simulink model "OPCModel"  (R2021a)
settings: Solver=VariableStepAuto  StartTime=0.0  StopTime=10.0  RelTol=1e-3
values from neighbouring files (symbols this model uses):
  ih = 22    [Data.m]
  it = 30    [Data.m]
  rhd = 0.75    [Data.m]
  rtd = 0.5    [Data.m]
undefined symbols (not defined in the file or in its folder): Ts
settings Model: Creator=jpss8  LastModifiedBy=jpss8

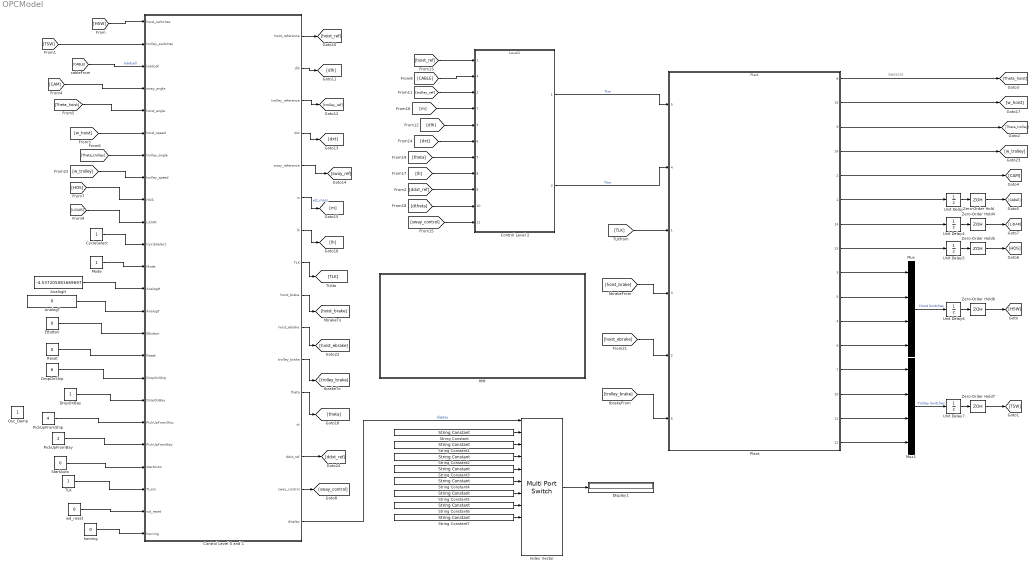
== system OPCModel ==
  note: Sensors
  AnalogH : Constant  Value=-4.537205081669697
  AnalogT : Constant  Value=0
  Control Level 0 and 1 : Subsystem
  Control Level 2 : ModelReference  ModelNameDialog=Level2.slx  SimulationMode=Normal  ModelReferenceVersion=1.293
      settings: PortSchema="{\"entries\":[{\"content\":{\"sides\":[{\"content\":{\"connectorIds\":[\"In1\",\"In4\",\"In2\",\"In7\",\"In3\",\"In6\",\"In5\",\"In8\",\"In9\",\"In10\",\"In11\"]},\"type\":\"ConnectorPlacement.EquallySpacedRectSide\",\"uuid\":\"5b552c0d-337f-40a2-963f-8f26f74218b0\"},{\"content\":{\"connectorIds\":[\"Out1\",\"Out2\"],\"side\":\"RIGHT\"},\"type\":\"ConnectorPlacement.EquallySpacedRectSide\",\"uuid\":\"4a33d29a-936e-4be9-945f-1937d64852b3\"},{\"content\":{\"connectorIds\":[],\"side\":\"TOP\"},\"type\":\"ConnectorPlacement.EquallySpacedRectSide\",\"uuid\":\"a706c8bd-7eef-4f34-a788-a1dec70d0973\"}]},\"type\":\"ConnectorPlacement.EquallySpacedConnector\",\"uuid\":\"61d5689b-6159-4c49-bed6-a66cde254875\"}],\"packageUris\":[\"http://schema.mathworks.com/mf0/Connector/R2020b\"],\"version\":\"1.0\"}"
  CycleSelect : Constant
  Display1 : Display
  DropOnBay : Constant
  DropOnShip : Constant  Value=6
  EButton : Constant  Value=0
  HMI : Subsystem
  Index Vector : MultiPortSwitch  DataPortOrder=Zero-based contiguous  Inputs=10  DataPortForDefault=Additional data port  DiagnosticForDefault=None  zeroidx=on
  Mode : Constant
  Mux : Mux
  Mux1 : Mux
  Osc_Damp : Constant
  PickUpFromBay : Constant  Value=2
  PickUpFromShip : Constant  Value=4
  Plant : ModelReference  ModelNameDialog=Plant.slx  SimulationMode=Normal  ModelReferenceVersion=1.224
      settings: PortSchema="{\"entries\":[{\"content\":{\"sides\":[{\"content\":{\"connectorIds\":[\"In5\",\"In4\",\"In1\",\"In3\",\"In2\",\"In6\"]},\"type\":\"ConnectorPlacement.EquallySpacedRectSide\",\"uuid\":\"21bb6514-2ae1-4e91-8ba8-0048b23f5eee\"},{\"content\":{\"connectorIds\":[\"Out8\",\"Out15\",\"Out9\",\"Out16\",\"Out2\",\"Out1\",\"Out14\",\"Out13\",\"Out3\",\"Out5\",\"Out4\",\"Out6\",\"Out7\",\"Out10\",\"Out11\",\"Out12\"],\"side\":\"RIGHT\"},\"type\":\"ConnectorPlacement.EquallySpacedRectSide\",\"uuid\":\"76781d7b-468f-4fab-8408-33b7b044b816\"},{\"content\":{\"connectorIds\":[],\"side\":\"TOP\"},\"type\":\"ConnectorPlacement.EquallySpacedRectSide\",\"uuid\":\"b4764fd0-dcaa-4ab7-bf15-0e4691eece23\"},{\"content\":{\"connectorIds\":[],\"side\":\"BOTTOM\"},\"type\":\"ConnectorPlacement.EquallySpacedRectSide\",\"uuid\":\"a33a5376-8a56-4d9a-a092-0a068881fa89\"}]},\"type\":\"ConnectorPlacement.EquallySpacedConnector\",\"uuid\":\"81ec6fbc-127c-46f8-9807-91263d11131f\"}],\"packageUris\":[\"http://schema.mathworks.com/mf0/Connector/R2020b\"],\"version\":\"1.0\"}"
  Reset : Constant  Value=0
  StartAuto : Constant  Value=0
  String Constant : StringConstant  String="\"Exit manual zone to perform automatic positioning\""
  String Constant1 : StringConstant  String="\"Automatic Positioning\""
  String Constant2 : StringConstant  String="\"Manually engage the container\""
  String Constant3 : StringConstant  String="\"Manually release the container\""
  String Constant4 : StringConstant  String="\"Manual\""
  String Constant5 : StringConstant  String="\"Standby\""
  String Constant6 : StringConstant  String="\"Homing\""
  String Constant7 : StringConstant  String="\"Mass Estimation\""
  TLK : Constant
  Unit Delay{,4..7} (5 alike) : UnitDelay  SampleTime=Ts  HasFrameUpgradeWarning=on
  Zero-Order Hold{,4..7} (5 alike) : ZeroOrderHold  SampleTime=Ts
  homing : Constant  Value=0
  wd_reset : Constant  Value=0
  wires:
  [trolley_brake] -> Plant/6
  [hoist_brake] -> Plant/3
  [hoist_ebrake] -> Plant/2
  [TLK] -> Plant/1
  Control Level 2/1 -> Plant/5  "Ttm"
  Control Level 2/2 -> Plant/4  "Thm"
  [lh] -> Control Level 2/8
  [m] -> Control Level 2/7
  [dlh] -> Control Level 2/3
  [trolley_ref] -> Control Level 2/2
  [hoist_ref] -> Control Level 2/1
  [theta] -> Control Level 2/5
  [CABLE] -> Control Level 2/4
  [dxt] -> Control Level 2/6
  [ddxt_ref] -> Control Level 2/9
  [sway_control] -> Control Level 2/11
  [dtheta] -> Control Level 2/10
  String Constant/1 -> Index Vector/2
  String Constant5/1 -> Index Vector/7
  String Constant3/1 -> Index Vector/5
  String Constant2/1 -> Index Vector/4
  Index Vector/1 -> Display1/1
  Control Level 0 and 1/16(display) -> Index Vector/1  "display"
  String Constant6/1 -> Index Vector/8
  String Constant1/1 -> Index Vector/3
  String Constant4/1 -> Index Vector/6
  String Constant7/1 -> Index Vector/9
  Unit Delay5/1 -> Zero-Order Hold5/1
  Zero-Order Hold7/1 -> [TSW]
  Unit Delay/1 -> Zero-Order Hold/1
  Plant/2 -> [CAM]
  Zero-Order Hold4/1 -> [LiDAR]
  Zero-Order Hold5/1 -> [HOS]
  Plant/3 -> Mux/1
  Mux1/1 -> Unit Delay7/1  "Trolley Switches"
  Plant/14 -> Unit Delay4/1
  Plant/6 -> Mux/4
  Plant/12 -> Mux1/4
  Plant/1 -> Unit Delay/1
  Plant/11 -> Mux1/3
  Zero-Order Hold/1 -> [CABLE]
  Plant/13 -> Unit Delay5/1
  Plant/8 -> [Theta_hoist]
  Plant/5 -> Mux/2
  Plant/9 -> [Theta_trolley]
  Unit Delay4/1 -> Zero-Order Hold4/1
  Mux/1 -> Unit Delay6/1  "Hoist Switches"
  Plant/7 -> Mux1/1
  Plant/16 -> [w_trolley]
  Plant/15 -> [w_hoist]
  Plant/10 -> Mux1/2
  Zero-Order Hold6/1 -> [HSW]
  Unit Delay7/1 -> Zero-Order Hold7/1
  Unit Delay6/1 -> Zero-Order Hold6/1
  Plant/4 -> Mux/3
  PickUpFromShip/1 -> Control Level 0 and 1/19(PickUpFromShip)
  wd_reset/1 -> Control Level 0 and 1/23(wd_reset)
  AnalogT/1 -> Control Level 0 and 1/14(AnalogT)
  EButton/1 -> Control Level 0 and 1/15(EButton)
  [Theta_hoist] -> Control Level 0 and 1/5(hoist_angle)
  StartAuto/1 -> Control Level 0 and 1/21(startAuto)
  TLK/1 -> Control Level 0 and 1/22(TLock)
  [LiDAR] -> Control Level 0 and 1/10(LiDAR)
  [Theta_trolley] -> Control Level 0 and 1/7(trolley_angle)
  [HOS] -> Control Level 0 and 1/9(HOS)
  DropOnBay/1 -> Control Level 0 and 1/18(DropOnBay)
  [HSW] -> Control Level 0 and 1/1(hoist_switches)
  CycleSelect/1 -> Control Level 0 and 1/11(CycleSelect)
  [CAM] -> Control Level 0 and 1/4(sway_angle)
  PickUpFromBay/1 -> Control Level 0 and 1/20(PickUpFromBay)
  [CABLE] -> Control Level 0 and 1/3(loadcell)  "loadcell"
  Mode/1 -> Control Level 0 and 1/12(Mode)
  [TSW] -> Control Level 0 and 1/2(trolley_switches)
  AnalogH/1 -> Control Level 0 and 1/13(AnalogH)
  DropOnShip/1 -> Control Level 0 and 1/17(DropOnShip)
  Reset/1 -> Control Level 0 and 1/16(Reset)
  Control Level 0 and 1/10(hoist_ebrake) -> [hoist_ebrake]
  Control Level 0 and 1/9(hoist_brake) -> [hoist_brake]
  Control Level 0 and 1/12(theta) -> [theta]
  Control Level 0 and 1/6(m) -> [m]  "est_mass"
  Control Level 0 and 1/7(lh) -> [lh]
  Control Level 0 and 1/5(sway_reference) -> [sway_ref]
  Control Level 0 and 1/8(TLK) -> [TLK]
  Control Level 0 and 1/2(dlh) -> [dlh]
  Control Level 0 and 1/4(dxt) -> [dxt]
  Control Level 0 and 1/3(trolley_reference) -> [trolley_ref]
  Control Level 0 and 1/11(trolley_brake) -> [trolley_brake]
  Control Level 0 and 1/1(hoist_reference) -> [hoist_ref]
  Control Level 0 and 1/14(ddxt_ref) -> [ddxt_ref]
  Control Level 0 and 1/15(sway_control) -> [sway_control]
  [w_hoist] -> Control Level 0 and 1/6(hoist_speed)
  [w_trolley] -> Control Level 0 and 1/8(trolley_speed)
  homing/1 -> Control Level 0 and 1/24(homing)

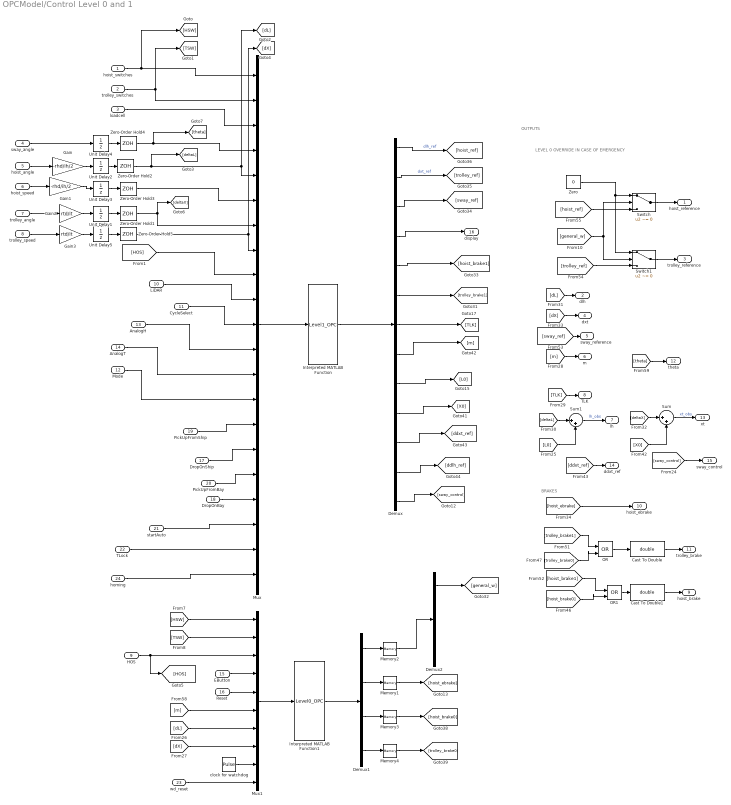
== system OPCModel/Control Level 0 and 1 ==
  note: LEVEL 0 OVERRIDE IN CASE OF EMERGENCY
  note: BRAKES
  note: OUTPUTS
  hoist_switches : Inport
  trolley_switches : Inport  Port=2
  loadcell : Inport  Port=3
  sway_angle : Inport  Port=4
  hoist_angle : Inport  Port=5
  hoist_speed : Inport  Port=6
  trolley_angle : Inport  Port=7
  trolley_speed : Inport  Port=8
  HOS : Inport  Port=9
  LiDAR : Inport  Port=10
  CycleSelect : Inport  Port=11
  Mode : Inport  Port=12
  AnalogH : Inport  Port=13
  AnalogT : Inport  Port=14
  EButton : Inport  Port=15
  Reset : Inport  Port=16
  DropOnShip : Inport  Port=17
  DropOnBay : Inport  Port=18
  PickUpFromShip : Inport  Port=19
  PickUpFromBay : Inport  Port=20
  startAuto : Inport  Port=21
  TLock : Inport  Port=22
  wd_reset : Inport  Port=23
  homing : Inport  Port=24
  Cast To Double : DataTypeConversion  OutDataTypeStr=double
  Cast To Double1 : DataTypeConversion  OutDataTypeStr=double
  Demux : Demux  Outputs=13
  Demux1 : Demux
  Demux2 : Demux
  Gain : Gain  Gain=-rhd/ih/2
  Gain1 : Gain  Gain=-rhd/ih/2
  Gain2 : Gain  Gain=rtd/it
  Gain3 : Gain  Gain=rtd/it
  Interpreted MATLAB Function : MATLABFcn  MATLABFcn=Level1_OPC  OutputDimensions=13
  Interpreted MATLAB Function1 : MATLABFcn  MATLABFcn=Level0_OPC  OutputDimensions=4
  Memory{1..4} (4 alike) : Memory
  Mux : Mux  Inputs=21
  Mux1 : Mux  Inputs=10
  OR : Logic  Operator=OR  IconShape=distinctive  AllPortsSameDT=off  OutDataTypeStr=boolean
  OR1 : Logic  Operator=OR  IconShape=distinctive  AllPortsSameDT=off  OutDataTypeStr=boolean
  Sum : Sum  Inputs=|++
  Sum1 : Sum  Inputs=|++
  Switch : Switch  Criteria=u2 ~= 0
  Switch1 : Switch  Criteria=u2 ~= 0
  Unit Delay{1..5} (5 alike) : UnitDelay  SampleTime=Ts  HasFrameUpgradeWarning=on
  Zero : Constant  Value=0  OutDataTypeStr=Inherit: Inherit via back propagation
  Zero-Order Hold{1..5} (5 alike) : ZeroOrderHold  SampleTime=Ts
  clock for watchdog : DiscretePulseGenerator  PulseType=Time based  Period=1  PulseWidth=50
  hoist_reference : Outport
  dlh : Outport  Port=2
  trolley_reference : Outport  Port=3
  dxt : Outport  Port=4
  sway_reference : Outport  Port=5
  m : Outport  Port=6
  lh : Outport  Port=7
  TLK : Outport  Port=8
  hoist_brake : Outport  Port=9
  hoist_ebrake : Outport  Port=10
  trolley_brake : Outport  Port=11
  theta : Outport  Port=12
  xt : Outport  Port=13
  ddxt_ref : Outport  Port=14
  sway_control : Outport  Port=15
  display : Outport  Port=16
  wires:
  Interpreted MATLAB Function/1 -> Demux/1
  trolley_switches/1 -> [TSW], Mux/2
  loadcell/1 -> Mux/3
  sway_angle/1 -> Unit Delay4/1
  hoist_angle/1 -> Gain/1
  LiDAR/1 -> Mux/10
  CycleSelect/1 -> Mux/11
  Mode/1 -> Mux/14
  AnalogH/1 -> Mux/12
  AnalogT/1 -> Mux/13
  DropOnShip/1 -> Mux/16
  DropOnBay/1 -> Mux/18
  PickUpFromShip/1 -> Mux/15
  PickUpFromBay/1 -> Mux/17
  startAuto/1 -> Mux/19
  TLock/1 -> Mux/20
  Mux/1 -> Interpreted MATLAB Function/1
  hoist_speed/1 -> Gain1/1
  trolley_speed/1 -> Gain3/1
  homing/1 -> Mux/21
  Unit Delay4/1 -> Zero-Order Hold4/1
  Unit Delay3/1 -> Zero-Order Hold3/1
  Unit Delay2/1 -> Zero-Order Hold2/1
  Zero-Order Hold4/1 -> [theta], Mux/4
  Zero-Order Hold2/1 -> [deltaL], [dL], Mux/5
  Zero-Order Hold3/1 -> Mux/6
  Unit Delay5/1 -> Zero-Order Hold5/1
  Unit Delay1/1 -> Zero-Order Hold1/1
  Zero-Order Hold1/1 -> [deltaX], Mux/7
  Zero-Order Hold5/1 -> [dX], Mux/8
  Gain1/1 -> Unit Delay3/1
  Gain/1 -> Unit Delay2/1
  Gain2/1 -> Unit Delay1/1
  Gain3/1 -> Unit Delay5/1
  [HSW] -> Mux1/1
  [TSW] -> Mux1/2
  HOS/1 -> [HOS], Mux1/3
  wd_reset/1 -> Mux1/10
  clock for watchdog/1 -> Mux1/9
  Mux1/1 -> Interpreted MATLAB Function1/1
  Interpreted MATLAB Function1/1 -> Demux1/1
  hoist_switches/1 -> [HSW], Mux/1
  EButton/1 -> Mux1/4
  Reset/1 -> Mux1/5
  [m] -> Mux1/6
  [dX] -> Mux1/8
  [dL] -> Mux1/7
  Demux1/1 -> Memory2/1
  Memory2/1 -> Demux2/1
  Demux1/2 -> Memory1/1
  Demux1/3 -> Memory3/1
  Demux1/4 -> Memory4/1
  Demux2/1 -> [general_w]
  Memory4/1 -> [trolley_brake0]
  Memory3/1 -> [hoist_brake0]
  Memory1/1 -> [hoist_ebrake]
  [HOS] -> Mux/9
  Demux/11 -> [ddxt_ref]
  Demux/12 -> [ddlh_ref]
  Demux/3 -> [sway_ref]
  Demux/7 -> [TLK]
  Demux/8 -> [m]
  Demux/1 -> [hoist_ref]  "dlh_ref"
  Demux/2 -> [trolley_ref]  "dxt_ref"
  Demux/5 -> [hoist_brake1]
  Demux/4 -> display/1
  Demux/9 -> [L0]
  Demux/6 -> [trolley_brake1]
  Demux/13 -> [sway_control]
  Demux/10 -> [X0]
  [sway_ref] -> sway_reference/1
  [deltaL] -> Sum1/1
  [trolley_ref] -> Switch1/3
  [hoist_ref] -> Switch/3
  [dX] -> dxt/1
  [trolley_brake1] -> OR/1
  [dL] -> dlh/1
  [m] -> m/1
  [general_w] -> Switch/2, Switch1/2
  Cast To Double/1 -> trolley_brake/1
  Switch1/1 -> trolley_reference/1
  OR1/1 -> Cast To Double1/1
  [ddxt_ref] -> ddxt_ref/1
  Sum/1 -> xt/1  "xt_obs"
  [TLK] -> TLK/1
  [hoist_brake0] -> OR1/2
  [theta] -> theta/1
  OR/1 -> Cast To Double/1
  [L0] -> Sum1/2
  [deltaX] -> Sum/1
  [X0] -> Sum/2
  [hoist_ebrake] -> hoist_ebrake/1
  [trolley_brake0] -> OR/2
  Cast To Double1/1 -> hoist_brake/1
  [hoist_brake1] -> OR1/1
  Sum1/1 -> lh/1  "lh_obs"
  Switch/1 -> hoist_reference/1
  [sway_control] -> sway_control/1
  Zero/1 -> Switch1/1, Switch/1
  trolley_angle/1 -> Gain2/1

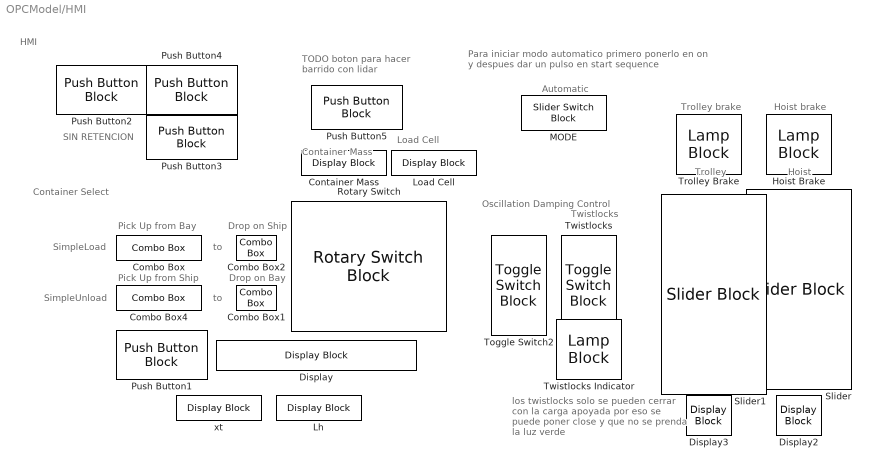
== system OPCModel/HMI ==
  note: los twistlocks solo se pueden cerrar con la carga apoyada
      | por eso se puede poner close y que no se prenda la luz verde
  note: Para iniciar modo automatico primero ponerlo en on y despues dar un pulso en start sequence
  note: TODO boton para hacer barrido con lidar
  note: SIN RETENCION
  note: Oscillation
      | Damping Control
  note: Container Select
  note: Trolley
  note: Automatic
  note: HMI
  note: Hoist
  note: Container Mass
  note: Pick Up from Ship
  note: Drop on Ship
  note: to
  note: to
  note: Drop on Bay
  note: Pick Up from Bay
  note: Twistlocks
  note: Trolley brake
  note: Hoist brake
  note: SimpleLoad
  note: SimpleUnload
  note: Load Cell
  Combo Box : ComboBox  LabelPosition=Hide  SelectedLabel=2
      settings: Values={{'1', '2', '3'}, [1 2 3]}
  Combo Box1 : ComboBox  LabelPosition=Hide  SelectedLabel=1
      settings: Values={{'1', '2', '3'}, [1 2 3]}
  Combo Box2 : ComboBox  LabelPosition=Hide  SelectedLabel=6
      settings: Values={{'1', '2', '3', '4', '5', '6', '7', '8', '9'}, [1 2 3 4 5 6 7 8 9]}
  Combo Box4 : ComboBox  LabelPosition=Hide  SelectedLabel=4
      settings: Values={{'1', '2', '3', '4', '5', '6', '7', '8', '9'}, [1 2 3 4 5 6 7 8 9]}
  Container Mass : DisplayBlock  LabelPosition=Hide  Format=short  Transparency=1
  Display : DisplayBlock  LabelPosition=Hide  Format=short  Alignment=Left  Transparency=1
  Display2 : DisplayBlock  LabelPosition=Hide  Format=short  Transparency=1
  Display3 : DisplayBlock  LabelPosition=Hide  Format=short  Transparency=1
  Hoist Brake : LampBlock  LabelPosition=Hide  Icon=Circle
  Lh : DisplayBlock  LabelPosition=Hide  Format=short  Transparency=1
  Load Cell : DisplayBlock  LabelPosition=Hide  Format=short  Transparency=1
  MODE : SliderSwitchBlock  LabelPosition=Hide
      settings: Values={{'On', 'Off'}, [1 0]}
  Push Button1 : PushButtonBlock  ButtonText=Start Sequence
  Push Button2 : PushButtonBlock  ButtonText=EMERGENCY
  Push Button3 : PushButtonBlock  ButtonText=RESET LEVEL0
  Push Button4 : PushButtonBlock  ButtonText=RESET WATCHDOG
  Push Button5 : PushButtonBlock  ButtonText=HOMING
  Rotary Switch : RotarySwitchBlock
      settings: Values={{'SimpleLoad', 'SimpleUnload', 'DoubleCycle'}, [1 2 3]}
  Slider : SliderBlock  LabelPosition=Hide  ScaleMin=-100  TickInterval=20
  Slider1 : SliderBlock  LabelPosition=Hide  ScaleMin=-100  TickInterval=20
  Toggle Switch2 : ToggleSwitchBlock  LabelPosition=Hide
      settings: Values={{'Off', 'On'}, [0 1]}
  Trolley Brake : LampBlock  LabelPosition=Hide  Icon=Circle
  Twistlocks : ToggleSwitchBlock  LabelPosition=Hide
      settings: Values={{'Close', 'Open'}, [1 0]}
  Twistlocks Indicator : LampBlock  LabelPosition=Hide  Icon=Circle
  xt : DisplayBlock  LabelPosition=Hide  Format=short  Transparency=1
